simulink model "servo"  (Simulink 4.00)
settings: Solver=ode45  StartTime=0.0  StopTime=2  RelTol=1e-3
InitFcn:
  | clear functions
libraries: truetime x1
settings Model: Creator=anton  LastModifiedBy=anton  OutputTimes=[0.00199]  LimitDataPoints=off  ExtModeTrigMode=oneshot  ExtModeArmWhenConnect=off  ExtModeAutoUpdateStatusClock=off  BlockReductionOpt=off

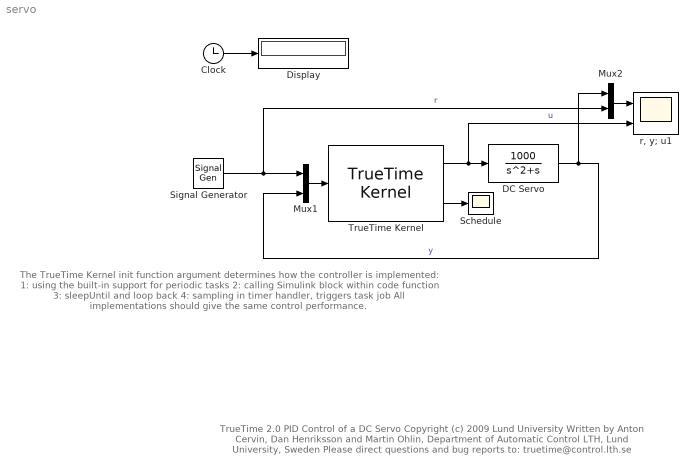
== system servo ==
  note: TrueTime 2.0  PID Control of a DC Servo
      | Copyright (c) 2009 Lund University
      | Written by Anton Cervin, Dan Henriksson and Martin Ohlin,
      | Department of Automatic Control LTH, Lund University, Sweden
      | Please direct questions and bug reports to: truetime@control.lth.se
  note: The TrueTime Kernel init function argument determines how the controller is implemented:
      |
      |   1: using the built-in support for periodic tasks
      |   2: calling Simulink block within code function
      |   3: sleepUntil and loop back
      |   4: sampling in timer handler, triggers task job
      |
      | All implementations should give the same control performance.
  Clock : Clock
      settings: DisplayTime=off  Decimation=10
  DC Servo : TransferFcn  Numerator=[1000]  Denominator=[1 1 0]  AbsoluteTolerance=auto  Realization=auto
  Display : Display
      settings: Format=short
  Mux1 : Mux  Inputs=2
  Mux2 : Mux  Inputs=2
  Schedule : Scope
      settings: TickLabels=on  TimeRange=2  YMin=0.8  YMax=1.7  SaveToWorkspace=off  SaveName=ScopeData2  DataFormat=Array  MaxDataPoints=5000
  Signal Generator : SignalGenerator  WaveForm=square  Amplitude=1  Frequency=1  Units=Hertz
  TrueTime Kernel : truetime/TrueTime Kernel  sfun=servo_init  args=1  ninputsoutputs=[2 1]  ntriggers=0  trigtype=falling  nwnodenbr=[]  clockoffsetdrift=[0 0]  schedoutput=on  battery=off  poweroutput=off
  "r, y; u1" : Scope  NumInputPorts=2
      settings: TimeRange=1  YMin=-1.5~-4  YMax=1.5~4  SaveToWorkspace=off  SaveName=y  MaxDataPoints=5000
  wires:
  TrueTime Kernel/1 -> DC Servo/1, "r, y; u1"/2  "u"
  Signal Generator/1 -> Mux1/1, Mux2/2  "r"
  Clock/1 -> Display/1
  DC Servo/1 -> Mux1/2, Mux2/1  "y"
  Mux1/1 -> TrueTime Kernel/1
  TrueTime Kernel/2 -> Schedule/1
  Mux2/1 -> "r, y; u1"/1
